simulink model "test"  (R2015a)
settings: Solver=ode45  StartTime=0.0  StopTime=380000  RelTol=1e-3
InitFcn:
  | %% DSPBuilder Start
  | alt_dspbuilder_update_model(bdroot)
  | %% DSPBuilder End
libraries: allblocks_alteradspbuilder2 x2155
(part 2 of 24)

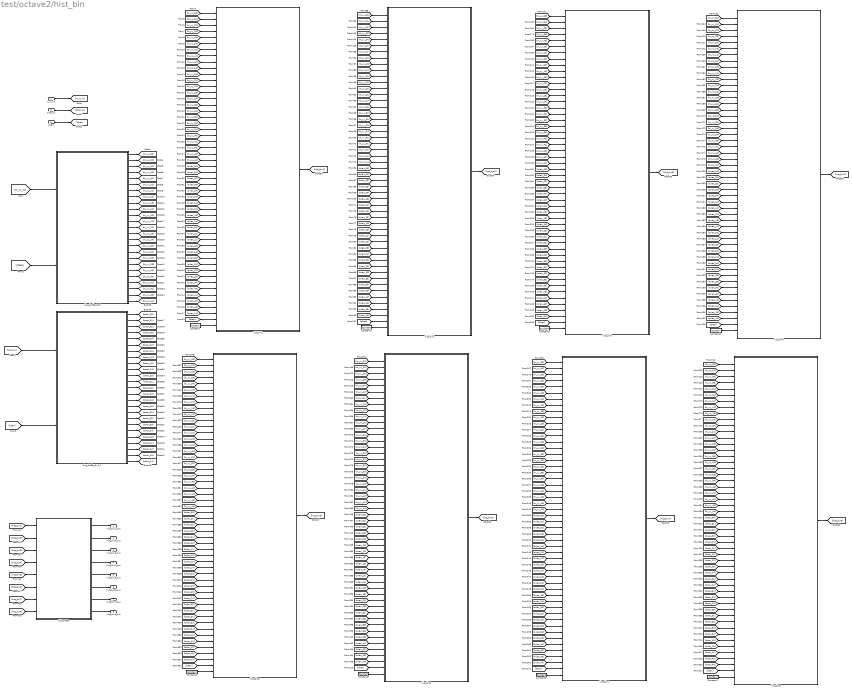
== system test/octave2/hist_bin ==
  m_xy_In : Inport
  orien_In : Inport  Port=2
  clken : Inport  Port=3
  Constant : allblocks_alteradspbuilder2/Constant  mask_cst=1  BusType=Unsigned Integer  bwl=8  bwr=0  roundMode=Truncate  satMode=Wrap  SpecifyClock=off  allowFloatingPointOverride=on  logOutputs=off  logFile=C:\Users\ASUS\Desktop\sift_fpga_final\Octave_2\tb_test\test_octave2_hist%5Fbin_Constant.fixedpointlog
  Constant1 : allblocks_alteradspbuilder2/Constant  mask_cst=2  BusType=Unsigned Integer  bwl=8  bwr=0  roundMode=Truncate  satMode=Wrap  SpecifyClock=off  allowFloatingPointOverride=on  logOutputs=off  logFile=C:\Users\ASUS\Desktop\sift_fpga_final\Octave_2\tb_test\test_octave2_hist%5Fbin_Constant1.fixedpointlog
  Constant2 : allblocks_alteradspbuilder2/Constant  mask_cst=3  BusType=Unsigned Integer  bwl=8  bwr=0  roundMode=Truncate  satMode=Wrap  SpecifyClock=off  allowFloatingPointOverride=on  logOutputs=off  logFile=C:\Users\ASUS\Desktop\sift_fpga_final\Octave_2\tb_test\test_octave2_hist%5Fbin_Constant2.fixedpointlog
  Constant3 : allblocks_alteradspbuilder2/Constant  mask_cst=4  BusType=Unsigned Integer  bwl=8  bwr=0  roundMode=Truncate  satMode=Wrap  SpecifyClock=off  allowFloatingPointOverride=on  logOutputs=off  logFile=C:\Users\ASUS\Desktop\sift_fpga_final\Octave_2\tb_test\test_octave2_hist%5Fbin_Constant3.fixedpointlog
  Constant4 : allblocks_alteradspbuilder2/Constant  mask_cst=5  BusType=Unsigned Integer  bwl=8  bwr=0  roundMode=Truncate  satMode=Wrap  SpecifyClock=off  allowFloatingPointOverride=on  logOutputs=off  logFile=C:\Users\ASUS\Desktop\sift_fpga_final\Octave_2\tb_test\test_octave2_hist%5Fbin_Constant4.fixedpointlog
  Constant5 : allblocks_alteradspbuilder2/Constant  mask_cst=6  BusType=Unsigned Integer  bwl=8  bwr=0  roundMode=Truncate  satMode=Wrap  SpecifyClock=off  allowFloatingPointOverride=on  logOutputs=off  logFile=C:\Users\ASUS\Desktop\sift_fpga_final\Octave_2\tb_test\test_octave2_hist%5Fbin_Constant5.fixedpointlog
  Constant6 : allblocks_alteradspbuilder2/Constant  mask_cst=7  BusType=Unsigned Integer  bwl=8  bwr=0  roundMode=Truncate  satMode=Wrap  SpecifyClock=off  allowFloatingPointOverride=on  logOutputs=off  logFile=C:\Users\ASUS\Desktop\sift_fpga_final\Octave_2\tb_test\test_octave2_hist%5Fbin_Constant6.fixedpointlog
  Constant7 : allblocks_alteradspbuilder2/Constant  mask_cst=8  BusType=Unsigned Integer  bwl=8  bwr=0  roundMode=Truncate  satMode=Wrap  SpecifyClock=off  allowFloatingPointOverride=on  logOutputs=off  logFile=C:\Users\ASUS\Desktop\sift_fpga_final\Octave_2\tb_test\test_octave2_hist%5Fbin_Constant7.fixedpointlog
  Line_buffer_5x5 : Subsystem
  Line_buffer_5x5_1 : Subsystem
  Subsystem : Subsystem
  hist_bin1 : Subsystem
  hist_bin2 : Subsystem
  hist_bin3 : Subsystem
  hist_bin4 : Subsystem
  hist_bin5 : Subsystem
  hist_bin6 : Subsystem
  hist_bin7 : Subsystem
  hist_bin8 : Subsystem
  hist_bin1_out : Outport
  hist_bin2_out : Outport  Port=2
  hist_bin3_out : Outport  Port=3
  hist_bin4_out : Outport  Port=4
  hist_bin5_out : Outport  Port=5
  hist_bin6_out : Outport  Port=6
  hist_bin7_out : Outport  Port=7
  hist_bin8_out : Outport  Port=8
  wires:
  [hist_bin7] -> Subsystem/7(hist_in_bin7)
  [m_xy_in] -> Line_buffer_5x5/1(dataIn)
  [clken] -> Line_buffer_5x5/2(clken)
  [clken] -> Line_buffer_5x5_1/2(clken)
  [orien_in] -> Line_buffer_5x5_1/1(dataIn)
  clken/1 -> [clken]
  Line_buffer_5x5_1/21(Out40) -> [orien_40]
  Line_buffer_5x5_1/19(Out33) -> [orien_33]
  Line_buffer_5x5_1/8(Out12) -> [orien_12]
  Line_buffer_5x5_1/14(Out23) -> [orien_23]
  Line_buffer_5x5_1/18(Out32) -> [orien_32]
  Line_buffer_5x5_1/20(Out34) -> [orien_34]
  Line_buffer_5x5_1/2(Out01) -> [orien_01]
  Line_buffer_5x5_1/7(Out11) -> [orien_11]
  Line_buffer_5x5_1/11(Out20) -> [orien_20]
  Line_buffer_5x5_1/13(Out22) -> [orien_22]
  Line_buffer_5x5_1/17(Out31) -> [orien_31]
  Line_buffer_5x5_1/25(Out44) -> [orien_44]
  Line_buffer_5x5_1/3(Out02) -> [orien_02]
  Line_buffer_5x5_1/5(Out04) -> [orien_04]
  Line_buffer_5x5_1/23(Out42) -> [orien_42]
  Line_buffer_5x5_1/24(Out43) -> [orien_43]
  Line_buffer_5x5_1/6(Out10) -> [orien_10]
  Line_buffer_5x5_1/1(Out00) -> [orien_00]
  Line_buffer_5x5_1/22(Out41) -> [orien_41]
  Line_buffer_5x5_1/15(Out24) -> [orien_24]
  Line_buffer_5x5_1/4(Out03) -> [orien_03]
  Line_buffer_5x5_1/9(Out13) -> [orien_13]
  Line_buffer_5x5_1/10(Out14) -> [orien_14]
  Line_buffer_5x5_1/12(Out21) -> [orien_21]
  Line_buffer_5x5_1/16(Out30) -> [orien_30]
  Line_buffer_5x5/24(Out43) -> [m_xy_43]
  Line_buffer_5x5/21(Out40) -> [m_xy_40]
  Line_buffer_5x5/23(Out42) -> [m_xy_42]
  Line_buffer_5x5/22(Out41) -> [m_xy_41]
  Line_buffer_5x5/25(Out44) -> [m_xy_44]
  Line_buffer_5x5/12(Out21) -> [m_xy_21]
  Line_buffer_5x5/15(Out24) -> [m_xy_24]
  Line_buffer_5x5/19(Out33) -> [m_xy_33]
  Line_buffer_5x5/18(Out32) -> [m_xy_32]
  Line_buffer_5x5/13(Out22) -> [m_xy_22]
  Line_buffer_5x5/11(Out20) -> [m_xy_20]
  Line_buffer_5x5/16(Out30) -> [m_xy_30]
  Line_buffer_5x5/14(Out23) -> [m_xy_23]
  Line_buffer_5x5/17(Out31) -> [m_xy_31]
  Line_buffer_5x5/20(Out34) -> [m_xy_34]
  [hist_bin1] -> Subsystem/1(hist_in_bin1)
  Line_buffer_5x5/1(Out00) -> [m_xy_00]
  [m_xy_04] -> hist_bin1/5(Mxy_In04)
  Line_buffer_5x5/2(Out01) -> [m_xy_01]
  hist_bin1/1(bin_out) -> [hist_bin1]
  [m_xy_10] -> hist_bin1/6(Mxy_In10)
  Line_buffer_5x5/9(Out13) -> [m_xy_13]
  [m_xy_13] -> hist_bin1/9(Mxy_In13)
  Line_buffer_5x5/10(Out14) -> [m_xy_14]
  Line_buffer_5x5/6(Out10) -> [m_xy_10]
  Line_buffer_5x5/7(Out11) -> [m_xy_11]
  [m_xy_11] -> hist_bin1/7(Mxy_In11)
  [m_xy_12] -> hist_bin1/8(Mxy_In12)
  Line_buffer_5x5/8(Out12) -> [m_xy_12]
  [m_xy_14] -> hist_bin1/10(Mxy_In14)
  [m_xy_22] -> hist_bin1/13(Mxy_In22)
  [m_xy_40] -> hist_bin1/21(Mxy_In40)
  [m_xy_43] -> hist_bin1/24(Mxy_In43)
  [m_xy_42] -> hist_bin1/23(Mxy_In42)
  [m_xy_44] -> hist_bin1/25(Mxy_In44)
  [m_xy_24] -> hist_bin1/15(Mxy_In24)
  [m_xy_21] -> hist_bin1/12(Mxy_In21)
  [m_xy_20] -> hist_bin1/11(Mxy_In20)
  [m_xy_23] -> hist_bin1/14(Mxy_In23)
  [m_xy_41] -> hist_bin1/22(Mxy_In41)
  [m_xy_01] -> hist_bin1/2(Mxy_In01)
  Line_buffer_5x5/4(Out03) -> [m_xy_03]
  Line_buffer_5x5/5(Out04) -> [m_xy_04]
  Line_buffer_5x5/3(Out02) -> [m_xy_02]
  [m_xy_31] -> hist_bin1/17(Mxy_In31)
  [m_xy_30] -> hist_bin1/16(Mxy_In30)
  [m_xy_34] -> hist_bin1/20(Mxy_In34)
  [m_xy_33] -> hist_bin1/19(Mxy_In33)
  [m_xy_32] -> hist_bin1/18(Mxy_In32)
  [m_xy_03] -> hist_bin1/4(Mxy_In03)
  [m_xy_02] -> hist_bin1/3(Mxy_In02)
  [hist_bin3] -> Subsystem/3(hist_in_bin3)
  [hist_bin4] -> Subsystem/4(hist_in_bin4)
  [orien_10] -> hist_bin1/31(Orien_In10)
  [orien_42] -> hist_bin1/48(Orien_In42)
  [orien_01] -> hist_bin1/27(Orien_In01)
  [orien_20] -> hist_bin1/36(Orien_In20)
  [orien_31] -> hist_bin1/42(Orien_In31)
  [orien_33] -> hist_bin1/44(Orien_In33)
  [orien_21] -> hist_bin1/37(Orien_In21)
  [orien_24] -> hist_bin1/40(Orien_In24)
  [orien_03] -> hist_bin1/29(Orien_In03)
  [orien_30] -> hist_bin1/41(Orien_In30)
  [orien_12] -> hist_bin1/33(Orien_In12)
  [orien_23] -> hist_bin1/39(Orien_In23)
  [orien_32] -> hist_bin1/43(Orien_In32)
  [orien_41] -> hist_bin1/47(Orien_In41)
  [orien_43] -> hist_bin1/49(Orien_In43)
  [orien_02] -> hist_bin1/28(Orien_In02)
  [orien_00] -> hist_bin1/26(Orien_In00)
  [orien_11] -> hist_bin1/32(Orien_In11)
  [orien_34] -> hist_bin1/45(Orien_In34)
  [orien_22] -> hist_bin1/38(Orien_In22)
  [orien_04] -> hist_bin1/30(Orien_In04)
  [orien_14] -> hist_bin1/35(Orien_In14)
  [orien_44] -> hist_bin1/50(Orien_In44)
  [orien_13] -> hist_bin1/34(Orien_In13)
  [orien_40] -> hist_bin1/46(Orien_In40)
  [clken] -> hist_bin1/51(clken)
  Constant/1 -> hist_bin1/52(bin_in)
  [m_xy_02] -> hist_bin2/3(Mxy_In02)
  [m_xy_04] -> hist_bin2/5(Mxy_In04)
  [m_xy_10] -> hist_bin2/6(Mxy_In10)
  [m_xy_23] -> hist_bin2/14(Mxy_In23)
  [m_xy_31] -> hist_bin2/17(Mxy_In31)
  [m_xy_30] -> hist_bin2/16(Mxy_In30)
  [m_xy_12] -> hist_bin2/8(Mxy_In12)
  [m_xy_32] -> hist_bin2/18(Mxy_In32)
  [m_xy_13] -> hist_bin2/9(Mxy_In13)
  [m_xy_33] -> hist_bin2/19(Mxy_In33)
  [m_xy_41] -> hist_bin2/22(Mxy_In41)
  [m_xy_01] -> hist_bin2/2(Mxy_In01)
  [m_xy_14] -> hist_bin2/10(Mxy_In14)
  [m_xy_40] -> hist_bin2/21(Mxy_In40)
  [m_xy_43] -> hist_bin2/24(Mxy_In43)
  [m_xy_20] -> hist_bin2/11(Mxy_In20)
  [m_xy_22] -> hist_bin2/13(Mxy_In22)
  [m_xy_24] -> hist_bin2/15(Mxy_In24)
  [m_xy_34] -> hist_bin2/20(Mxy_In34)
  [m_xy_03] -> hist_bin2/4(Mxy_In03)
  [m_xy_00] -> hist_bin2/1(Mxy_In00)
  [m_xy_11] -> hist_bin2/7(Mxy_In11)
  [m_xy_21] -> hist_bin2/12(Mxy_In21)
  [orien_31] -> hist_bin2/42(Orien_In31)
  [orien_34] -> hist_bin2/45(Orien_In34)
  [m_xy_42] -> hist_bin2/23(Mxy_In42)
  [orien_01] -> hist_bin2/27(Orien_In01)
  [orien_00] -> hist_bin2/26(Orien_In00)
  [orien_04] -> hist_bin2/30(Orien_In04)
  [orien_13] -> hist_bin2/34(Orien_In13)
  [orien_20] -> hist_bin2/36(Orien_In20)
  [orien_24] -> hist_bin2/40(Orien_In24)
  [orien_33] -> hist_bin2/44(Orien_In33)
  [orien_32] -> hist_bin2/43(Orien_In32)
  [orien_41] -> hist_bin2/47(Orien_In41)
  [orien_11] -> hist_bin2/32(Orien_In11)
  [orien_21] -> hist_bin2/37(Orien_In21)
  [orien_14] -> hist_bin2/35(Orien_In14)
  [orien_22] -> hist_bin2/38(Orien_In22)
  [orien_23] -> hist_bin2/39(Orien_In23)
  [orien_02] -> hist_bin2/28(Orien_In02)
  [orien_10] -> hist_bin2/31(Orien_In10)
  [orien_12] -> hist_bin2/33(Orien_In12)
  [orien_30] -> hist_bin2/41(Orien_In30)
  [m_xy_44] -> hist_bin2/25(Mxy_In44)
  [orien_03] -> hist_bin2/29(Orien_In03)
  [orien_40] -> hist_bin2/46(Orien_In40)
  [clken] -> hist_bin2/51(clken)
  hist_bin2/1(bin_out) -> [hist_bin2]
  [orien_42] -> hist_bin2/48(Orien_In42)
  [orien_44] -> hist_bin2/50(Orien_In44)
  [orien_43] -> hist_bin2/49(Orien_In43)
  Constant1/1 -> hist_bin2/52(bin_in)
  [m_xy_00] -> hist_bin1/1(Mxy_In00)
  Subsystem/4(bin4_out) -> hist_bin4_out/1
  Subsystem/3(bin3_out) -> hist_bin3_out/1
  [hist_bin8] -> Subsystem/8(hist_in_bin8)
  [hist_bin6] -> Subsystem/6(hist_in_bin6)
  [hist_bin5] -> Subsystem/5(hist_in_bin5)
  Subsystem/2(bin2_out) -> hist_bin2_out/1
  orien_In/1 -> [orien_in]
  m_xy_In/1 -> [m_xy_in]
  Subsystem/5(bin5_out) -> hist_bin5_out/1
  Subsystem/6(bin6_out) -> hist_bin6_out/1
  Subsystem/7(bin7_out) -> hist_bin7_out/1
  Subsystem/8(bin8_out) -> hist_bin8_out/1
  [hist_bin2] -> Subsystem/2(hist_in_bin2)
  [m_xy_04] -> hist_bin3/5(Mxy_In04)
  hist_bin3/1(bin_out) -> [hist_bin3]
  [m_xy_10] -> hist_bin3/6(Mxy_In10)
  [m_xy_13] -> hist_bin3/9(Mxy_In13)
  [m_xy_11] -> hist_bin3/7(Mxy_In11)
  [m_xy_12] -> hist_bin3/8(Mxy_In12)
  [m_xy_14] -> hist_bin3/10(Mxy_In14)
  [m_xy_22] -> hist_bin3/13(Mxy_In22)
  [m_xy_40] -> hist_bin3/21(Mxy_In40)
  [m_xy_43] -> hist_bin3/24(Mxy_In43)
  [m_xy_42] -> hist_bin3/23(Mxy_In42)
  [m_xy_44] -> hist_bin3/25(Mxy_In44)
  [m_xy_24] -> hist_bin3/15(Mxy_In24)
  [m_xy_21] -> hist_bin3/12(Mxy_In21)
  [m_xy_20] -> hist_bin3/11(Mxy_In20)
  [m_xy_23] -> hist_bin3/14(Mxy_In23)
  [m_xy_41] -> hist_bin3/22(Mxy_In41)
  [m_xy_01] -> hist_bin3/2(Mxy_In01)
  [m_xy_31] -> hist_bin3/17(Mxy_In31)
  [m_xy_30] -> hist_bin3/16(Mxy_In30)
  [m_xy_34] -> hist_bin3/20(Mxy_In34)
  [m_xy_33] -> hist_bin3/19(Mxy_In33)
  [m_xy_32] -> hist_bin3/18(Mxy_In32)
  [m_xy_03] -> hist_bin3/4(Mxy_In03)
  [m_xy_02] -> hist_bin3/3(Mxy_In02)
  [orien_10] -> hist_bin3/31(Orien_In10)
  [orien_42] -> hist_bin3/48(Orien_In42)
  [orien_01] -> hist_bin3/27(Orien_In01)
  [orien_20] -> hist_bin3/36(Orien_In20)
  [orien_31] -> hist_bin3/42(Orien_In31)
  [orien_33] -> hist_bin3/44(Orien_In33)
  [orien_21] -> hist_bin3/37(Orien_In21)
  [orien_24] -> hist_bin3/40(Orien_In24)
  [orien_03] -> hist_bin3/29(Orien_In03)
  [orien_30] -> hist_bin3/41(Orien_In30)
  [orien_12] -> hist_bin3/33(Orien_In12)
  [orien_23] -> hist_bin3/39(Orien_In23)
  [orien_32] -> hist_bin3/43(Orien_In32)
  [orien_41] -> hist_bin3/47(Orien_In41)
  [orien_43] -> hist_bin3/49(Orien_In43)
  [orien_02] -> hist_bin3/28(Orien_In02)
  [orien_00] -> hist_bin3/26(Orien_In00)
  [orien_11] -> hist_bin3/32(Orien_In11)
  [orien_34] -> hist_bin3/45(Orien_In34)
  [orien_22] -> hist_bin3/38(Orien_In22)
  [orien_04] -> hist_bin3/30(Orien_In04)
  [orien_14] -> hist_bin3/35(Orien_In14)
  [orien_44] -> hist_bin3/50(Orien_In44)
  [orien_13] -> hist_bin3/34(Orien_In13)
  [orien_40] -> hist_bin3/46(Orien_In40)
  [clken] -> hist_bin3/51(clken)
  Constant2/1 -> hist_bin3/52(bin_in)
  [m_xy_02] -> hist_bin4/3(Mxy_In02)
  [m_xy_04] -> hist_bin4/5(Mxy_In04)
  [m_xy_10] -> hist_bin4/6(Mxy_In10)
  [m_xy_23] -> hist_bin4/14(Mxy_In23)
  [m_xy_31] -> hist_bin4/17(Mxy_In31)
  [m_xy_30] -> hist_bin4/16(Mxy_In30)
  [m_xy_12] -> hist_bin4/8(Mxy_In12)
  [m_xy_32] -> hist_bin4/18(Mxy_In32)
  [m_xy_13] -> hist_bin4/9(Mxy_In13)
  [m_xy_33] -> hist_bin4/19(Mxy_In33)
  [m_xy_41] -> hist_bin4/22(Mxy_In41)
  [m_xy_01] -> hist_bin4/2(Mxy_In01)
  [m_xy_14] -> hist_bin4/10(Mxy_In14)
  [m_xy_40] -> hist_bin4/21(Mxy_In40)
  [m_xy_43] -> hist_bin4/24(Mxy_In43)
  [m_xy_20] -> hist_bin4/11(Mxy_In20)
  [m_xy_22] -> hist_bin4/13(Mxy_In22)
  [m_xy_24] -> hist_bin4/15(Mxy_In24)
  [m_xy_34] -> hist_bin4/20(Mxy_In34)
  [m_xy_03] -> hist_bin4/4(Mxy_In03)
  [m_xy_00] -> hist_bin4/1(Mxy_In00)
  [m_xy_11] -> hist_bin4/7(Mxy_In11)
  [m_xy_21] -> hist_bin4/12(Mxy_In21)
  [orien_31] -> hist_bin4/42(Orien_In31)
  [orien_34] -> hist_bin4/45(Orien_In34)
  [m_xy_42] -> hist_bin4/23(Mxy_In42)
  [orien_01] -> hist_bin4/27(Orien_In01)
  [orien_00] -> hist_bin4/26(Orien_In00)
  [orien_04] -> hist_bin4/30(Orien_In04)
  [orien_13] -> hist_bin4/34(Orien_In13)
  [orien_20] -> hist_bin4/36(Orien_In20)
  [orien_24] -> hist_bin4/40(Orien_In24)
  [orien_33] -> hist_bin4/44(Orien_In33)
  [orien_32] -> hist_bin4/43(Orien_In32)
  [orien_41] -> hist_bin4/47(Orien_In41)
  [orien_11] -> hist_bin4/32(Orien_In11)
  [orien_21] -> hist_bin4/37(Orien_In21)
  [orien_14] -> hist_bin4/35(Orien_In14)
  [orien_22] -> hist_bin4/38(Orien_In22)
  [orien_23] -> hist_bin4/39(Orien_In23)
  [orien_02] -> hist_bin4/28(Orien_In02)
  [orien_10] -> hist_bin4/31(Orien_In10)
  [orien_12] -> hist_bin4/33(Orien_In12)
  [orien_30] -> hist_bin4/41(Orien_In30)
  [m_xy_44] -> hist_bin4/25(Mxy_In44)
  [orien_03] -> hist_bin4/29(Orien_In03)
  [orien_40] -> hist_bin4/46(Orien_In40)
  [clken] -> hist_bin4/51(clken)
  hist_bin4/1(bin_out) -> [hist_bin4]
  [orien_42] -> hist_bin4/48(Orien_In42)
  [orien_44] -> hist_bin4/50(Orien_In44)
  [orien_43] -> hist_bin4/49(Orien_In43)
  Constant3/1 -> hist_bin4/52(bin_in)
  [m_xy_00] -> hist_bin3/1(Mxy_In00)
  [m_xy_04] -> hist_bin5/5(Mxy_In04)
  hist_bin5/1(bin_out) -> [hist_bin5]
  [m_xy_10] -> hist_bin5/6(Mxy_In10)
  [m_xy_13] -> hist_bin5/9(Mxy_In13)
  [m_xy_11] -> hist_bin5/7(Mxy_In11)
  [m_xy_12] -> hist_bin5/8(Mxy_In12)
  [m_xy_14] -> hist_bin5/10(Mxy_In14)
  [m_xy_22] -> hist_bin5/13(Mxy_In22)
  [m_xy_40] -> hist_bin5/21(Mxy_In40)
  [m_xy_43] -> hist_bin5/24(Mxy_In43)
  [m_xy_42] -> hist_bin5/23(Mxy_In42)
  [m_xy_44] -> hist_bin5/25(Mxy_In44)
  [m_xy_24] -> hist_bin5/15(Mxy_In24)
  [m_xy_21] -> hist_bin5/12(Mxy_In21)
  [m_xy_20] -> hist_bin5/11(Mxy_In20)
  [m_xy_23] -> hist_bin5/14(Mxy_In23)
  [m_xy_41] -> hist_bin5/22(Mxy_In41)
  [m_xy_01] -> hist_bin5/2(Mxy_In01)
  [m_xy_31] -> hist_bin5/17(Mxy_In31)
  [m_xy_30] -> hist_bin5/16(Mxy_In30)
  [m_xy_34] -> hist_bin5/20(Mxy_In34)
  [m_xy_33] -> hist_bin5/19(Mxy_In33)
  [m_xy_32] -> hist_bin5/18(Mxy_In32)
  [m_xy_03] -> hist_bin5/4(Mxy_In03)
  [m_xy_02] -> hist_bin5/3(Mxy_In02)
  [orien_10] -> hist_bin5/31(Orien_In10)
  [orien_42] -> hist_bin5/48(Orien_In42)
  [orien_01] -> hist_bin5/27(Orien_In01)
  [orien_20] -> hist_bin5/36(Orien_In20)
  [orien_31] -> hist_bin5/42(Orien_In31)
  [orien_33] -> hist_bin5/44(Orien_In33)
  [orien_21] -> hist_bin5/37(Orien_In21)
  [orien_24] -> hist_bin5/40(Orien_In24)
  [orien_03] -> hist_bin5/29(Orien_In03)
  [orien_30] -> hist_bin5/41(Orien_In30)
  [orien_12] -> hist_bin5/33(Orien_In12)
  [orien_23] -> hist_bin5/39(Orien_In23)
  [orien_32] -> hist_bin5/43(Orien_In32)
  [orien_41] -> hist_bin5/47(Orien_In41)
  [orien_43] -> hist_bin5/49(Orien_In43)
  [orien_02] -> hist_bin5/28(Orien_In02)
  [orien_00] -> hist_bin5/26(Orien_In00)
  [orien_11] -> hist_bin5/32(Orien_In11)
  [orien_34] -> hist_bin5/45(Orien_In34)
  [orien_22] -> hist_bin5/38(Orien_In22)
  [orien_04] -> hist_bin5/30(Orien_In04)
  [orien_14] -> hist_bin5/35(Orien_In14)
  [orien_44] -> hist_bin5/50(Orien_In44)
  [orien_13] -> hist_bin5/34(Orien_In13)
  [orien_40] -> hist_bin5/46(Orien_In40)
  [clken] -> hist_bin5/51(clken)
  Constant4/1 -> hist_bin5/52(bin_in)
  [m_xy_02] -> hist_bin6/3(Mxy_In02)
  [m_xy_04] -> hist_bin6/5(Mxy_In04)
  [m_xy_10] -> hist_bin6/6(Mxy_In10)
  [m_xy_23] -> hist_bin6/14(Mxy_In23)
  [m_xy_31] -> hist_bin6/17(Mxy_In31)
  [m_xy_30] -> hist_bin6/16(Mxy_In30)
  [m_xy_12] -> hist_bin6/8(Mxy_In12)
  [m_xy_32] -> hist_bin6/18(Mxy_In32)
  [m_xy_13] -> hist_bin6/9(Mxy_In13)
  [m_xy_33] -> hist_bin6/19(Mxy_In33)
  [m_xy_41] -> hist_bin6/22(Mxy_In41)
  [m_xy_01] -> hist_bin6/2(Mxy_In01)
  [m_xy_14] -> hist_bin6/10(Mxy_In14)
  [m_xy_40] -> hist_bin6/21(Mxy_In40)
  [m_xy_43] -> hist_bin6/24(Mxy_In43)
  [m_xy_20] -> hist_bin6/11(Mxy_In20)
  [m_xy_22] -> hist_bin6/13(Mxy_In22)
  [m_xy_24] -> hist_bin6/15(Mxy_In24)
  [m_xy_34] -> hist_bin6/20(Mxy_In34)
  [m_xy_03] -> hist_bin6/4(Mxy_In03)
  [m_xy_00] -> hist_bin6/1(Mxy_In00)
  [m_xy_11] -> hist_bin6/7(Mxy_In11)
  [m_xy_21] -> hist_bin6/12(Mxy_In21)
  [orien_31] -> hist_bin6/42(Orien_In31)
  [orien_34] -> hist_bin6/45(Orien_In34)
  [m_xy_42] -> hist_bin6/23(Mxy_In42)
  [orien_01] -> hist_bin6/27(Orien_In01)
  [orien_00] -> hist_bin6/26(Orien_In00)
  [orien_04] -> hist_bin6/30(Orien_In04)
  [orien_13] -> hist_bin6/34(Orien_In13)
  [orien_20] -> hist_bin6/36(Orien_In20)
  [orien_24] -> hist_bin6/40(Orien_In24)
  [orien_33] -> hist_bin6/44(Orien_In33)
  [orien_32] -> hist_bin6/43(Orien_In32)
  [orien_41] -> hist_bin6/47(Orien_In41)
  [orien_11] -> hist_bin6/32(Orien_In11)
  [orien_21] -> hist_bin6/37(Orien_In21)
  [orien_14] -> hist_bin6/35(Orien_In14)
  [orien_22] -> hist_bin6/38(Orien_In22)
  [orien_23] -> hist_bin6/39(Orien_In23)
  [orien_02] -> hist_bin6/28(Orien_In02)
  [orien_10] -> hist_bin6/31(Orien_In10)
  [orien_12] -> hist_bin6/33(Orien_In12)
  [orien_30] -> hist_bin6/41(Orien_In30)
  [m_xy_44] -> hist_bin6/25(Mxy_In44)
  [orien_03] -> hist_bin6/29(Orien_In03)
  [orien_40] -> hist_bin6/46(Orien_In40)
  [clken] -> hist_bin6/51(clken)
  hist_bin6/1(bin_out) -> [hist_bin6]
  [orien_42] -> hist_bin6/48(Orien_In42)
  [orien_44] -> hist_bin6/50(Orien_In44)
  [orien_43] -> hist_bin6/49(Orien_In43)
  Constant5/1 -> hist_bin6/52(bin_in)
  [m_xy_00] -> hist_bin5/1(Mxy_In00)
  [m_xy_04] -> hist_bin7/5(Mxy_In04)
  hist_bin7/1(bin_out) -> [hist_bin7]
  [m_xy_10] -> hist_bin7/6(Mxy_In10)
  [m_xy_13] -> hist_bin7/9(Mxy_In13)
  [m_xy_11] -> hist_bin7/7(Mxy_In11)
  [m_xy_12] -> hist_bin7/8(Mxy_In12)
  [m_xy_14] -> hist_bin7/10(Mxy_In14)
  [m_xy_22] -> hist_bin7/13(Mxy_In22)
  [m_xy_40] -> hist_bin7/21(Mxy_In40)
  [m_xy_43] -> hist_bin7/24(Mxy_In43)
  [m_xy_42] -> hist_bin7/23(Mxy_In42)
  [m_xy_44] -> hist_bin7/25(Mxy_In44)
  [m_xy_24] -> hist_bin7/15(Mxy_In24)
  [m_xy_21] -> hist_bin7/12(Mxy_In21)
  [m_xy_20] -> hist_bin7/11(Mxy_In20)
  [m_xy_23] -> hist_bin7/14(Mxy_In23)
  [m_xy_41] -> hist_bin7/22(Mxy_In41)
  [m_xy_01] -> hist_bin7/2(Mxy_In01)
  [m_xy_31] -> hist_bin7/17(Mxy_In31)
  [m_xy_30] -> hist_bin7/16(Mxy_In30)
  [m_xy_34] -> hist_bin7/20(Mxy_In34)
  [m_xy_33] -> hist_bin7/19(Mxy_In33)
  [m_xy_32] -> hist_bin7/18(Mxy_In32)
  [m_xy_03] -> hist_bin7/4(Mxy_In03)
  [m_xy_02] -> hist_bin7/3(Mxy_In02)
  [orien_10] -> hist_bin7/31(Orien_In10)
  [orien_42] -> hist_bin7/48(Orien_In42)
  [orien_01] -> hist_bin7/27(Orien_In01)
  [orien_20] -> hist_bin7/36(Orien_In20)
  [orien_31] -> hist_bin7/42(Orien_In31)
  [orien_33] -> hist_bin7/44(Orien_In33)
  [orien_21] -> hist_bin7/37(Orien_In21)
  [orien_24] -> hist_bin7/40(Orien_In24)
  [orien_03] -> hist_bin7/29(Orien_In03)
  [orien_30] -> hist_bin7/41(Orien_In30)
  [orien_12] -> hist_bin7/33(Orien_In12)
  [orien_23] -> hist_bin7/39(Orien_In23)
  [orien_32] -> hist_bin7/43(Orien_In32)
  [orien_41] -> hist_bin7/47(Orien_In41)
  [orien_43] -> hist_bin7/49(Orien_In43)
  [orien_02] -> hist_bin7/28(Orien_In02)
  [orien_00] -> hist_bin7/26(Orien_In00)
  [orien_11] -> hist_bin7/32(Orien_In11)
  [orien_34] -> hist_bin7/45(Orien_In34)
  [orien_22] -> hist_bin7/38(Orien_In22)
  [orien_04] -> hist_bin7/30(Orien_In04)
  [orien_14] -> hist_bin7/35(Orien_In14)
  [orien_44] -> hist_bin7/50(Orien_In44)
  [orien_13] -> hist_bin7/34(Orien_In13)
  [orien_40] -> hist_bin7/46(Orien_In40)
  [clken] -> hist_bin7/51(clken)
  Constant6/1 -> hist_bin7/52(bin_in)
  [m_xy_02] -> hist_bin8/3(Mxy_In02)
  [m_xy_04] -> hist_bin8/5(Mxy_In04)
  [m_xy_10] -> hist_bin8/6(Mxy_In10)
  [m_xy_23] -> hist_bin8/14(Mxy_In23)
  [m_xy_31] -> hist_bin8/17(Mxy_In31)
  [m_xy_30] -> hist_bin8/16(Mxy_In30)
  [m_xy_12] -> hist_bin8/8(Mxy_In12)
  [m_xy_32] -> hist_bin8/18(Mxy_In32)
  [m_xy_13] -> hist_bin8/9(Mxy_In13)
  [m_xy_33] -> hist_bin8/19(Mxy_In33)
  [m_xy_41] -> hist_bin8/22(Mxy_In41)
  [m_xy_01] -> hist_bin8/2(Mxy_In01)
  [m_xy_14] -> hist_bin8/10(Mxy_In14)
  [m_xy_40] -> hist_bin8/21(Mxy_In40)
  [m_xy_43] -> hist_bin8/24(Mxy_In43)
  [m_xy_20] -> hist_bin8/11(Mxy_In20)
  [m_xy_22] -> hist_bin8/13(Mxy_In22)
  [m_xy_24] -> hist_bin8/15(Mxy_In24)
  [m_xy_34] -> hist_bin8/20(Mxy_In34)
  [m_xy_03] -> hist_bin8/4(Mxy_In03)
  [m_xy_00] -> hist_bin8/1(Mxy_In00)
  [m_xy_11] -> hist_bin8/7(Mxy_In11)
  [m_xy_21] -> hist_bin8/12(Mxy_In21)
  [orien_31] -> hist_bin8/42(Orien_In31)
  [orien_34] -> hist_bin8/45(Orien_In34)
  [m_xy_42] -> hist_bin8/23(Mxy_In42)
  [orien_01] -> hist_bin8/27(Orien_In01)
  [orien_00] -> hist_bin8/26(Orien_In00)
  [orien_04] -> hist_bin8/30(Orien_In04)
  [orien_13] -> hist_bin8/34(Orien_In13)
  [orien_20] -> hist_bin8/36(Orien_In20)
  [orien_24] -> hist_bin8/40(Orien_In24)
  [orien_33] -> hist_bin8/44(Orien_In33)
  [orien_32] -> hist_bin8/43(Orien_In32)
  [orien_41] -> hist_bin8/47(Orien_In41)
  [orien_11] -> hist_bin8/32(Orien_In11)
  [orien_21] -> hist_bin8/37(Orien_In21)
  [orien_14] -> hist_bin8/35(Orien_In14)
  [orien_22] -> hist_bin8/38(Orien_In22)
  [orien_23] -> hist_bin8/39(Orien_In23)
  [orien_02] -> hist_bin8/28(Orien_In02)
  [orien_10] -> hist_bin8/31(Orien_In10)
  [orien_12] -> hist_bin8/33(Orien_In12)
  [orien_30] -> hist_bin8/41(Orien_In30)
  [m_xy_44] -> hist_bin8/25(Mxy_In44)
  [orien_03] -> hist_bin8/29(Orien_In03)
  [orien_40] -> hist_bin8/46(Orien_In40)
  [clken] -> hist_bin8/51(clken)
  hist_bin8/1(bin_out) -> [hist_bin8]
  [orien_42] -> hist_bin8/48(Orien_In42)
  [orien_44] -> hist_bin8/50(Orien_In44)
  [orien_43] -> hist_bin8/49(Orien_In43)
  Constant7/1 -> hist_bin8/52(bin_in)
  [m_xy_00] -> hist_bin7/1(Mxy_In00)
  Subsystem/1(bin1_out) -> hist_bin1_out/1

== system test/octave2/scale_space ==
  data_in : Inport
  valid_in : Inport  Port=2
  Gaussian_scale1 : Subsystem
  Gaussian_scale2 : Subsystem
  Gaussian_scale3 : Subsystem
  Gaussian_scale4 : Subsystem
  scale4 : Outport
  scale3 : Outport  Port=2
  scale2 : Outport  Port=3
  scale1 : Outport  Port=4
  wires:
  data_in/1 -> [pixel_in]
  valid_in/1 -> [valid_in]
  [pixel_in] -> Gaussian_scale3/1(pixel_in)
  [pixel_in] -> Gaussian_scale4/1(pixel_in)
  [valid_in] -> Gaussian_scale3/2(valid_in)
  [pixel_in] -> Gaussian_scale1/1(pixel_in)
  [valid_in] -> Gaussian_scale1/2(valid_in)
  [valid_in] -> Gaussian_scale4/2(valid_in)
  [pixel_in] -> Gaussian_scale2/1(pixel_in)
  [valid_in] -> Gaussian_scale2/2(valid_in)
  Gaussian_scale3/1(pixel_out) -> [pixel_scale3]
  [pixel_scale3] -> scale3/1
  [pixel_scale2] -> scale2/1
  Gaussian_scale4/1(pixel_out) -> [pixel_scale4]
  [pixel_scale4] -> scale4/1
  Gaussian_scale1/1(pixel_out) -> [pixel_scale1]
  Gaussian_scale2/1(pixel_out) -> [pixel_scale2]
  [pixel_scale1] -> scale1/1

== system test/octave2/GradOrien/lineBuff_3x3 ==
  dataIn : Inport
  clken : Inport  Port=2
  Delay : allblocks_alteradspbuilder2/Delay  pipeline=1  pipeline_display=1  ClockPhase=1  use_ena=on  use_sclr=off  allowFloatingPointOverride=on  logOutputs=off  logFile=C:\Users\ASUS\Desktop\sift_fpga_final\Octave_2\tb_test\test_octave2_GradOrien_lineBuff%5F3x3_Delay.fixedpointlog  use_init=off  reset_value=1
  Delay1 : allblocks_alteradspbuilder2/Delay  pipeline=1  pipeline_display=1  ClockPhase=1  use_ena=on  use_sclr=off  allowFloatingPointOverride=on  logOutputs=off  logFile=C:\Users\ASUS\Desktop\sift_fpga_final\Octave_2\tb_test\test_octave2_GradOrien_lineBuff%5F3x3_Delay1.fixedpointlog  use_init=off  reset_value=1
  Delay2 : allblocks_alteradspbuilder2/Delay  pipeline=1  pipeline_display=1  ClockPhase=1  use_ena=on  use_sclr=off  allowFloatingPointOverride=on  logOutputs=off  logFile=C:\Users\ASUS\Desktop\sift_fpga_final\Octave_2\tb_test\test_octave2_GradOrien_lineBuff%5F3x3_Delay2.fixedpointlog  use_init=off  reset_value=1
  Delay5 : allblocks_alteradspbuilder2/Delay  pipeline=1  pipeline_display=1  ClockPhase=1  use_ena=on  use_sclr=off  allowFloatingPointOverride=on  logOutputs=off  logFile=C:\Users\ASUS\Desktop\sift_fpga_final\Octave_2\tb_test\test_octave2_GradOrien_lineBuff%5F3x3_Delay5.fixedpointlog  use_init=off  reset_value=1
  Delay6 : allblocks_alteradspbuilder2/Delay  pipeline=1  pipeline_display=1  ClockPhase=1  use_ena=on  use_sclr=off  allowFloatingPointOverride=on  logOutputs=off  logFile=C:\Users\ASUS\Desktop\sift_fpga_final\Octave_2\tb_test\test_octave2_GradOrien_lineBuff%5F3x3_Delay6.fixedpointlog  use_init=off  reset_value=1
  Delay9 : allblocks_alteradspbuilder2/Delay  pipeline=1  pipeline_display=1  ClockPhase=1  use_ena=on  use_sclr=off  allowFloatingPointOverride=on  logOutputs=off  logFile=C:\Users\ASUS\Desktop\sift_fpga_final\Octave_2\tb_test\test_octave2_GradOrien_lineBuff%5F3x3_Delay9.fixedpointlog  use_init=off  reset_value=1
  Memory Delay : allblocks_alteradspbuilder2/Memory Delay  BusType=Signed Fractional  bwl=9  bwr=16  pipeline=638  pipeline_display=638  ram_type=AUTO  use_ena=on  use_sclr=off  allowFloatingPointOverride=on  logOutputs=off  logFile=C:\Users\ASUS\Desktop\sift_fpga_final\Octave_2\tb_test\test_octave2_GradOrien_lineBuff%5F3x3_Memory+Delay.fixedpointlog
  Memory Delay1 : allblocks_alteradspbuilder2/Memory Delay  BusType=Signed Fractional  bwl=9  bwr=16  pipeline=638  pipeline_display=638  ram_type=AUTO  use_ena=on  use_sclr=off  allowFloatingPointOverride=on  logOutputs=off  logFile=C:\Users\ASUS\Desktop\sift_fpga_final\Octave_2\tb_test\test_octave2_GradOrien_lineBuff%5F3x3_Memory+Delay1.fixedpointlog
  To Workspace : ToWorkspace  VariableName=data_in1  SaveFormat=Timeseries  SampleTime=-1
  To Workspace1 : ToWorkspace  VariableName=data_in2  SaveFormat=Timeseries  SampleTime=-1
  Out01 : Outport
  Out10 : Outport  Port=2
  Out12 : Outport  Port=3
  Out21 : Outport  Port=4
  wires:
  Delay1/1 -> [data_01], Delay2/1
  [clken] -> Memory Delay1/2
  Delay6/1 -> Memory Delay1/1, [data_12]
  Memory Delay1/1 -> Delay9/1
  [clken] -> Delay9/2
  [clken] -> Delay1/2
  [clken] -> Delay/2
  [data_in] -> To Workspace/1, Delay/1
  [clken] -> Delay2/2
  Delay2/1 -> Memory Delay/1
  clken/1 -> [clken]
  [data_21] -> Out21/1
  [data_10] -> Out10/1
  Memory Delay/1 -> [data_10], Delay5/1
  [clken] -> Memory Delay/2
  [clken] -> Delay6/2
  Delay5/1 -> Delay6/1
  [data_12] -> Out12/1
  [data_01] -> Out01/1
  [clken] -> Delay5/2
  dataIn/1 -> [data_in]
  Delay9/1 -> [data_21]
  Delay/1 -> To Workspace1/1, Delay1/1

== system test/octave2/GradOrien/sub_GradOrian ==
  L_y_add_1 : Inport
  L_x_add_1 : Inport  Port=2
  L_x_sub_1 : Inport  Port=3
  L_y_sub_1 : Inport  Port=4
  clken : Inport  Port=5
  AltBus : allblocks_alteradspbuilder2/AltBus  BusType=Unsigned Integer  bwl=10  bwr=0  saturate=off  floatingPointInput=on  floatingPointOutput=on  logOutputs=off  logFile=C:\Users\ASUS\Desktop\sift_fpga_final\Octave_2\tb_test\test_octave2_GradOrien_sub%5FGradOrian_AltBus.fixedpointlog
  Bus Builder : allblocks_alteradspbuilder2/Bus Builder  BusType=Unsigned Integer  bwl=3  bwr=1  pipeline_display=0
  Comparator3 : allblocks_alteradspbuilder2/Comparator  direction=a > b  pipeline_display=0  allowFloatingPointOverride=on  logOutputs=off  logFile=C:\Users\ASUS\Desktop\sift_fpga_final\Octave_2\tb_test\test_octave2_GradOrien_sub%5FGradOrian_Comparator3.fixedpointlog
  Comparator4 : allblocks_alteradspbuilder2/Comparator  direction=a > b  pipeline_display=0  allowFloatingPointOverride=on  logOutputs=off  logFile=C:\Users\ASUS\Desktop\sift_fpga_final\Octave_2\tb_test\test_octave2_GradOrien_sub%5FGradOrian_Comparator4.fixedpointlog
  Comparator5 : allblocks_alteradspbuilder2/Comparator  direction=a > b  pipeline_display=0  allowFloatingPointOverride=on  logOutputs=off  logFile=C:\Users\ASUS\Desktop\sift_fpga_final\Octave_2\tb_test\test_octave2_GradOrien_sub%5FGradOrian_Comparator5.fixedpointlog
  Constant : allblocks_alteradspbuilder2/Constant  mask_cst=5  BusType=Unsigned Integer  bwl=8  bwr=0  roundMode=Truncate  satMode=Wrap  SpecifyClock=off  allowFloatingPointOverride=on  logOutputs=off  logFile=C:\Users\ASUS\Desktop\sift_fpga_final\Octave_2\tb_test\test_octave2_GradOrien_sub%5FGradOrian_Constant.fixedpointlog
  Constant1 : allblocks_alteradspbuilder2/Constant  mask_cst=4  BusType=Unsigned Integer  bwl=8  bwr=0  roundMode=Truncate  satMode=Wrap  SpecifyClock=off  allowFloatingPointOverride=on  logOutputs=off  logFile=C:\Users\ASUS\Desktop\sift_fpga_final\Octave_2\tb_test\test_octave2_GradOrien_sub%5FGradOrian_Constant1.fixedpointlog
  Constant2 : allblocks_alteradspbuilder2/Constant  mask_cst=7  BusType=Unsigned Integer  bwl=8  bwr=0  roundMode=Truncate  satMode=Wrap  SpecifyClock=off  allowFloatingPointOverride=on  logOutputs=off  logFile=C:\Users\ASUS\Desktop\sift_fpga_final\Octave_2\tb_test\test_octave2_GradOrien_sub%5FGradOrian_Constant2.fixedpointlog
  Constant3 : allblocks_alteradspbuilder2/Constant  mask_cst=1  BusType=Unsigned Integer  bwl=8  bwr=0  roundMode=Truncate  satMode=Wrap  SpecifyClock=off  allowFloatingPointOverride=on  logOutputs=off  logFile=C:\Users\ASUS\Desktop\sift_fpga_final\Octave_2\tb_test\test_octave2_GradOrien_sub%5FGradOrian_Constant3.fixedpointlog
  Constant4 : allblocks_alteradspbuilder2/Constant  mask_cst=6  BusType=Unsigned Integer  bwl=8  bwr=0  roundMode=Truncate  satMode=Wrap  SpecifyClock=off  allowFloatingPointOverride=on  logOutputs=off  logFile=C:\Users\ASUS\Desktop\sift_fpga_final\Octave_2\tb_test\test_octave2_GradOrien_sub%5FGradOrian_Constant4.fixedpointlog
  Constant5 : allblocks_alteradspbuilder2/Constant  mask_cst=3  BusType=Unsigned Integer  bwl=8  bwr=0  roundMode=Truncate  satMode=Wrap  SpecifyClock=off  allowFloatingPointOverride=on  logOutputs=off  logFile=C:\Users\ASUS\Desktop\sift_fpga_final\Octave_2\tb_test\test_octave2_GradOrien_sub%5FGradOrian_Constant5.fixedpointlog
  Constant6 : allblocks_alteradspbuilder2/Constant  mask_cst=8  BusType=Unsigned Integer  bwl=8  bwr=0  roundMode=Truncate  satMode=Wrap  SpecifyClock=off  allowFloatingPointOverride=on  logOutputs=off  logFile=C:\Users\ASUS\Desktop\sift_fpga_final\Octave_2\tb_test\test_octave2_GradOrien_sub%5FGradOrian_Constant6.fixedpointlog
  Constant7 : allblocks_alteradspbuilder2/Constant  mask_cst=2  BusType=Unsigned Integer  bwl=8  bwr=0  roundMode=Truncate  satMode=Wrap  SpecifyClock=off  allowFloatingPointOverride=on  logOutputs=off  logFile=C:\Users\ASUS\Desktop\sift_fpga_final\Octave_2\tb_test\test_octave2_GradOrien_sub%5FGradOrian_Constant7.fixedpointlog
  Delay : allblocks_alteradspbuilder2/Delay  pipeline=1  pipeline_display=1  ClockPhase=1  use_ena=on  use_sclr=off  allowFloatingPointOverride=on  logOutputs=off  logFile=C:\Users\ASUS\Desktop\sift_fpga_final\Octave_2\tb_test\test_octave2_GradOrien_sub%5FGradOrian_Delay.fixedpointlog  use_init=off  reset_value=1
  Delay1 : allblocks_alteradspbuilder2/Delay  pipeline=1  pipeline_display=1  ClockPhase=1  use_ena=on  use_sclr=off  allowFloatingPointOverride=on  logOutputs=off  logFile=C:\Users\ASUS\Desktop\sift_fpga_final\Octave_2\tb_test\test_octave2_GradOrien_sub%5FGradOrian_Delay1.fixedpointlog  use_init=off  reset_value=1
  Delay2 : allblocks_alteradspbuilder2/Delay  pipeline=1  pipeline_display=1  ClockPhase=1  use_ena=on  use_sclr=off  allowFloatingPointOverride=on  logOutputs=off  logFile=C:\Users\ASUS\Desktop\sift_fpga_final\Octave_2\tb_test\test_octave2_GradOrien_sub%5FGradOrian_Delay2.fixedpointlog  use_init=off  reset_value=1
  Multiplexer2 : allblocks_alteradspbuilder2/Multiplexer  numInputs=8  pipeline=0  oneHot=off  pipeline_display=0  use_ena=off  use_aclr=off  allowFloatingPointOverride=on  logOutputs=off  logFile=C:\Users\ASUS\Desktop\sift_fpga_final\Octave_2\tb_test\test_octave2_GradOrien_sub%5FGradOrian_Multiplexer2.fixedpointlog
  Multiplexer3 : allblocks_alteradspbuilder2/Multiplexer  numInputs=2  pipeline=0  oneHot=off  pipeline_display=0  use_ena=off  use_aclr=off  allowFloatingPointOverride=on  logOutputs=off  logFile=C:\Users\ASUS\Desktop\sift_fpga_final\Octave_2\tb_test\test_octave2_GradOrien_sub%5FGradOrian_Multiplexer3.fixedpointlog
  Multiplexer4 : allblocks_alteradspbuilder2/Multiplexer  numInputs=2  pipeline=0  oneHot=off  pipeline_display=0  use_ena=off  use_aclr=off  allowFloatingPointOverride=on  logOutputs=off  logFile=C:\Users\ASUS\Desktop\sift_fpga_final\Octave_2\tb_test\test_octave2_GradOrien_sub%5FGradOrian_Multiplexer4.fixedpointlog
  Parallel Adder Subtractor : allblocks_alteradspbuilder2/Parallel Adder Subtractor  number_of_inputs=2  direction=+-  use_pipeline=on  pipeline_display=1  phase_selection=1  use_ena=on  use_aclr=off  allowFloatingPointOverride=on  logOutputs=off  logFile=C:\Users\ASUS\Desktop\sift_fpga_final\Octave_2\tb_test\test_octave2_GradOrien_sub%5FGradOrian_Parallel+Adder+Subtractor.fixedpointlog
  Parallel Adder Subtractor1 : allblocks_alteradspbuilder2/Parallel Adder Subtractor  number_of_inputs=2  direction=+-  use_pipeline=on  pipeline_display=1  phase_selection=1  use_ena=on  use_aclr=off  allowFloatingPointOverride=on  logOutputs=off  logFile=C:\Users\ASUS\Desktop\sift_fpga_final\Octave_2\tb_test\test_octave2_GradOrien_sub%5FGradOrian_Parallel+Adder+Subtractor1.fixedpointlog
  Parallel Adder Subtractor2 : allblocks_alteradspbuilder2/Parallel Adder Subtractor  number_of_inputs=2  direction=-+  use_pipeline=on  pipeline_display=1  phase_selection=1  use_ena=on  use_aclr=off  allowFloatingPointOverride=on  logOutputs=off  logFile=C:\Users\ASUS\Desktop\sift_fpga_final\Octave_2\tb_test\test_octave2_GradOrien_sub%5FGradOrian_Parallel+Adder+Subtractor2.fixedpointlog
  Parallel Adder Subtractor3 : allblocks_alteradspbuilder2/Parallel Adder Subtractor  number_of_inputs=2  direction=-+  use_pipeline=on  pipeline_display=1  phase_selection=1  use_ena=on  use_aclr=off  allowFloatingPointOverride=on  logOutputs=off  logFile=C:\Users\ASUS\Desktop\sift_fpga_final\Octave_2\tb_test\test_octave2_GradOrien_sub%5FGradOrian_Parallel+Adder+Subtractor3.fixedpointlog
  Parallel Adder Subtractor5 : allblocks_alteradspbuilder2/Parallel Adder Subtractor  number_of_inputs=2  direction=++  use_pipeline=on  pipeline_display=1  phase_selection=1  use_ena=on  use_aclr=off  allowFloatingPointOverride=on  logOutputs=off  logFile=C:\Users\ASUS\Desktop\sift_fpga_final\Octave_2\tb_test\test_octave2_GradOrien_sub%5FGradOrian_Parallel+Adder+Subtractor5.fixedpointlog
  To Workspace : ToWorkspace  VariableName=mxy  SaveFormat=Timeseries  SampleTime=-1
  To Workspace1 : ToWorkspace  VariableName=orien  SaveFormat=Timeseries  SampleTime=-1
  orien : Outport
  m_xy : Outport  Port=2
  wires:
  Multiplexer2/1 -> Delay2/1
  Bus Builder/1 -> Multiplexer2/1
  Constant6/1 -> Multiplexer2/8
  Constant4/1 -> Multiplexer2/6
  Constant5/1 -> Multiplexer2/7
  Comparator3/1 -> Delay/1
  Constant7/1 -> Multiplexer2/9
  [L_y_sub_1] -> Comparator4/2
  [L_x_sub_1] -> Comparator3/2
  [L_y_add_1] -> Comparator4/1
  [L_x_add_1] -> Comparator3/1
  [Ly_1] -> Multiplexer4/2
  Delay1/1 -> Bus Builder/2, Multiplexer4/1
  [Lx] -> Multiplexer3/3
  Delay/1 -> Bus Builder/1, Multiplexer3/1
  [Lx_1] -> Multiplexer3/2
  [Ly] -> Multiplexer4/3
  Constant/1 -> Multiplexer2/2
  [clken] -> Delay1/2
  Comparator5/1 -> Bus Builder/3
  [clken] -> Delay/2
  Comparator4/1 -> Delay1/1
  Multiplexer4/1 -> Comparator5/2, Parallel Adder Subtractor5/2
  Multiplexer3/1 -> Comparator5/1, Parallel Adder Subtractor5/1
  [clken] -> Parallel Adder Subtractor5/3
  [clken] -> Delay2/2
  Constant1/1 -> Multiplexer2/3
  Parallel Adder Subtractor2/1 -> [Lx_1]
  [clken] -> Parallel Adder Subtractor2/3
  [L_y_add_1] -> Parallel Adder Subtractor3/1
  Parallel Adder Subtractor3/1 -> [Ly_1]
  [L_y_sub_1] -> Parallel Adder Subtractor3/2
  [L_x_sub_1] -> Parallel Adder Subtractor2/2
  [clken] -> Parallel Adder Subtractor3/3
  [L_x_add_1] -> Parallel Adder Subtractor2/1
  [L_x_sub_1] -> Parallel Adder Subtractor/2
  [L_y_sub_1] -> Parallel Adder Subtractor1/2
  [L_y_add_1] -> Parallel Adder Subtractor1/1
  [clken] -> Parallel Adder Subtractor/3
  Parallel Adder Subtractor/1 -> [Lx]
  Parallel Adder Subtractor1/1 -> [Ly]
  [clken] -> Parallel Adder Subtractor1/3
  [L_x_add_1] -> Parallel Adder Subtractor/1
  Constant2/1 -> Multiplexer2/4
  Constant3/1 -> Multiplexer2/5
  L_x_add_1/1 -> [L_x_add_1]
  L_x_sub_1/1 -> [L_x_sub_1]
  L_y_add_1/1 -> [L_y_add_1]
  L_y_sub_1/1 -> [L_y_sub_1]
  AltBus/1 -> m_xy/1
  clken/1 -> [clken]
  Parallel Adder Subtractor5/1 -> To Workspace/1, AltBus/1
  Delay2/1 -> To Workspace1/1, orien/1

== system test/octave2/Ram/Subsystem ==
  descriptor : Inport
  eof : Inport  Port=2
  AltBus : allblocks_alteradspbuilder2/AltBus  BusType=Single Bit  bwl=8  bwr=0  saturate=off  floatingPointInput=on  floatingPointOutput=on  logOutputs=off  logFile=C:\Users\ASUS\Desktop\sift_fpga_final\Octave_2\tb_test\test_octave2_Ram_Subsystem_AltBus.fixedpointlog
  AltBus1 : allblocks_alteradspbuilder2/AltBus  BusType=Unsigned Integer  bwl=1172  bwr=0  saturate=off  floatingPointInput=on  floatingPointOutput=on  logOutputs=off  logFile=C:\Users\ASUS\Desktop\sift_fpga_final\Octave_2\tb_test\test_octave2_Ram_Subsystem_AltBus1.fixedpointlog
  Counter : allblocks_alteradspbuilder2/Counter  BusType=Unsigned Integer  bwl=10  bwr=0  use_modulo=on  modulo=1000  SpecifyClock=off  direction=Increment  use_sload=off  use_sset=off  svalue=1  use_clk_ena=off  use_ena=on  use_sclr=on  pipeline_display=1
  Logical Bus Operator : allblocks_alteradspbuilder2/Logical Bus Operator  BusType=Unsigned Integer  bwl=1173  bwr=0  LogicalOp_text=Shift Right  mask_value_num=-5  shift_amount=1172  force_sign_ext=off  pipeline_display=0
  data : Outport
  add_write : Outport  Port=2
  ena_write : Outport  Port=3
  wires:
  descriptor/1 -> [descriptor]
  [descriptor] -> Logical Bus Operator/1
  Logical Bus Operator/1 -> AltBus/1
  AltBus/1 -> [isKeyPoint]
  [isKeyPoint] -> Counter/1
  eof/1 -> [eof]
  [eof] -> Counter/2
  Counter/1 -> [add_write]
  [add_write] -> add_write/1
  [isKeyPoint] -> ena_write/1
  [descriptor] -> AltBus1/1
  AltBus1/1 -> [data]
  [data] -> data/1

== system test/octave2/Ram/Subsystem1 ==
  descriptor : Inport
  eof : Inport  Port=2
  AltBus : allblocks_alteradspbuilder2/AltBus  BusType=Single Bit  bwl=8  bwr=0  saturate=off  floatingPointInput=on  floatingPointOutput=on  logOutputs=off  logFile=C:\Users\ASUS\Desktop\sift_fpga_final\Octave_2\tb_test\test_octave2_Ram_Subsystem1_AltBus.fixedpointlog
  AltBus1 : allblocks_alteradspbuilder2/AltBus  BusType=Unsigned Integer  bwl=1172  bwr=0  saturate=off  floatingPointInput=on  floatingPointOutput=on  logOutputs=off  logFile=C:\Users\ASUS\Desktop\sift_fpga_final\Octave_2\tb_test\test_octave2_Ram_Subsystem1_AltBus1.fixedpointlog
  Counter : allblocks_alteradspbuilder2/Counter  BusType=Unsigned Integer  bwl=10  bwr=0  use_modulo=on  modulo=1000  SpecifyClock=off  direction=Increment  use_sload=off  use_sset=off  svalue=1  use_clk_ena=off  use_ena=on  use_sclr=on  pipeline_display=1
  Logical Bus Operator : allblocks_alteradspbuilder2/Logical Bus Operator  BusType=Unsigned Integer  bwl=1173  bwr=0  LogicalOp_text=Shift Right  mask_value_num=-5  shift_amount=1172  force_sign_ext=off  pipeline_display=0
  data : Outport
  add_write : Outport  Port=2
  ena_write : Outport  Port=3
  wires:
  descriptor/1 -> [descriptor]
  [descriptor] -> Logical Bus Operator/1
  Logical Bus Operator/1 -> AltBus/1
  AltBus/1 -> [isKeyPoint]
  [isKeyPoint] -> Counter/1
  eof/1 -> [eof]
  [eof] -> Counter/2
  Counter/1 -> [add_write]
  [add_write] -> add_write/1
  [isKeyPoint] -> ena_write/1
  [descriptor] -> AltBus1/1
  AltBus1/1 -> [data]
  [data] -> data/1

== system test/octave2/calculate_key_point/find_KeyPoint ==
  dataIn_10 : Inport
  dataIn_11 : Inport  Port=2
  dataIn_12 : Inport  Port=3
  dataIn_13 : Inport  Port=4
  dataIn_14 : Inport  Port=5
  dataIn_15 : Inport  Port=6
  dataIn_16 : Inport  Port=7
  dataIn_17 : Inport  Port=8
  dataIn_18 : Inport  Port=9
  dataIn_20 : Inport  Port=10
  dataIn_21 : Inport  Port=11
  dataIn_22 : Inport  Port=12
  dataIn_23 : Inport  Port=13
  dataIn_24 : Inport  Port=14
  dataIn_25 : Inport  Port=15
  dataIn_26 : Inport  Port=16
  dataIn_27 : Inport  Port=17
  dataIn_28 : Inport  Port=18
  dataIn_30 : Inport  Port=19
  dataIn_31 : Inport  Port=20
  dataIn_32 : Inport  Port=21
  dataIn_33 : Inport  Port=22
  dataIn_34 : Inport  Port=23
  dataIn_35 : Inport  Port=24
  dataIn_36 : Inport  Port=25
  dataIn_37 : Inport  Port=26
  dataIn_38 : Inport  Port=27
  Logical Bit Operator : allblocks_alteradspbuilder2/Logical Bit Operator  LogicalOperator=OR  user_inputs=2  pipeline_display=0
  find_Keymax : Subsystem
  find_min : Subsystem
  is_KeyPoint : Outport
  wires:
  [dataIn_32] -> find_Keymax/21(dataIn_32)
  [dataIn_33] -> find_Keymax/22(dataIn_33)
  [dataIn_36] -> find_Keymax/25(dataIn_36)
  [dataIn_37] -> find_Keymax/26(dataIn_37)
  [dataIn_34] -> find_Keymax/23(dataIn_34)
  [dataIn_35] -> find_Keymax/24(dataIn_35)
  [dataIn_30] -> find_Keymax/19(dataIn_30)
  [dataIn_31] -> find_Keymax/20(dataIn_31)
  [is_KeyPoint_Max] -> Logical Bit Operator/2
  [is_KeyPoint_Min] -> Logical Bit Operator/1
  find_Keymax/1(is_KeyPoint) -> [is_KeyPoint_Max]
  [dataIn_28] -> find_Keymax/18(dataIn_28)
  [dataIn_26] -> find_Keymax/16(dataIn_26)
  [dataIn_22] -> find_Keymax/12(dataIn_22)
  [dataIn_27] -> find_Keymax/17(dataIn_27)
  [dataIn_20] -> find_Keymax/10(dataIn_20)
  [dataIn_23] -> find_Keymax/13(dataIn_23)
  [dataIn_24] -> find_Keymax/14(dataIn_24)
  [dataIn_21] -> find_Keymax/11(dataIn_21)
  [dataIn_25] -> find_Keymax/15(dataIn_25)
  [dataIn_10] -> find_Keymax/1(dataIn_10)
  [dataIn_11] -> find_Keymax/2(dataIn_11)
  [dataIn_12] -> find_Keymax/3(dataIn_12)
  dataIn_23/1 -> [dataIn_23]
  dataIn_17/1 -> [dataIn_17]
  dataIn_22/1 -> [dataIn_22]
  dataIn_14/1 -> [dataIn_14]
  dataIn_16/1 -> [dataIn_16]
  dataIn_28/1 -> [dataIn_28]
  dataIn_20/1 -> [dataIn_20]
  dataIn_21/1 -> [dataIn_21]
  dataIn_26/1 -> [dataIn_26]
  dataIn_10/1 -> [dataIn_10]
  dataIn_30/1 -> [dataIn_30]
  dataIn_27/1 -> [dataIn_27]
  dataIn_25/1 -> [dataIn_25]
  dataIn_15/1 -> [dataIn_15]
  dataIn_18/1 -> [dataIn_18]
  dataIn_24/1 -> [dataIn_24]
  dataIn_32/1 -> [dataIn_32]
  dataIn_13/1 -> [dataIn_13]
  dataIn_31/1 -> [dataIn_31]
  [dataIn_14] -> find_Keymax/5(dataIn_14)
  dataIn_34/1 -> [dataIn_34]
  dataIn_11/1 -> [dataIn_11]
  [dataIn_17] -> find_Keymax/8(dataIn_17)
  dataIn_35/1 -> [dataIn_35]
  dataIn_33/1 -> [dataIn_33]
  dataIn_38/1 -> [dataIn_38]
  [dataIn_13] -> find_Keymax/4(dataIn_13)
  [dataIn_16] -> find_Keymax/7(dataIn_16)
  [dataIn_15] -> find_Keymax/6(dataIn_15)
  dataIn_12/1 -> [dataIn_12]
  [dataIn_18] -> find_Keymax/9(dataIn_18)
  dataIn_36/1 -> [dataIn_36]
  dataIn_37/1 -> [dataIn_37]
  [dataIn_38] -> find_Keymax/27(dataIn_38)
  find_min/1(is_KeyPoint) -> [is_KeyPoint_Min]
  [dataIn_11] -> find_min/2(dataIn_11)
  [dataIn_12] -> find_min/3(dataIn_12)
  [dataIn_13] -> find_min/4(dataIn_13)
  [dataIn_15] -> find_min/6(dataIn_15)
  [dataIn_16] -> find_min/7(dataIn_16)
  [dataIn_17] -> find_min/8(dataIn_17)
  [dataIn_18] -> find_min/9(dataIn_18)
  [dataIn_31] -> find_min/20(dataIn_31)
  [dataIn_14] -> find_min/5(dataIn_14)
  [is_KeyPoint] -> is_KeyPoint/1
  [dataIn_33] -> find_min/22(dataIn_33)
  [dataIn_32] -> find_min/21(dataIn_32)
  [dataIn_34] -> find_min/23(dataIn_34)
  [dataIn_35] -> find_min/24(dataIn_35)
  [dataIn_36] -> find_min/25(dataIn_36)
  [dataIn_21] -> find_min/11(dataIn_21)
  [dataIn_22] -> find_min/12(dataIn_22)
  [dataIn_23] -> find_min/13(dataIn_23)
  [dataIn_25] -> find_min/15(dataIn_25)
  [dataIn_24] -> find_min/14(dataIn_24)
  [dataIn_38] -> find_min/27(dataIn_38)
  [dataIn_20] -> find_min/10(dataIn_20)
  [dataIn_26] -> find_min/16(dataIn_26)
  [dataIn_30] -> find_min/19(dataIn_30)
  [dataIn_27] -> find_min/17(dataIn_27)
  [dataIn_37] -> find_min/26(dataIn_37)
  [dataIn_28] -> find_min/18(dataIn_28)
  [dataIn_10] -> find_min/1(dataIn_10)
  Logical Bit Operator/1 -> [is_KeyPoint]
